simulink model "FTSMC"  (R2022b)
settings: Solver=FixedStepAuto  StartTime=0.0  StopTime=3  FixedStep=1e-5  RelTol=1e-3
libraries: spsSeriesRLCBranchLib x4, spsStairGeneratorLib x3, spsControlledVoltageSourceLib x2, spsCurrentMeasurementLib x2, spsDiodeLib x2, spsIGBTLib x2, spsVariableResistorLib x2, spsVoltageMeasurementLib x2, slpidlib x1, spspowerguiLib x1
settings Model: Creator=10721  LastModifiedBy=10721

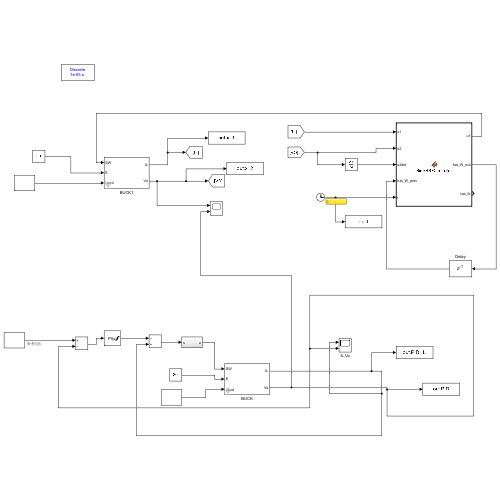
[thumbnail: Simulink's stored preview of the top-level diagram]
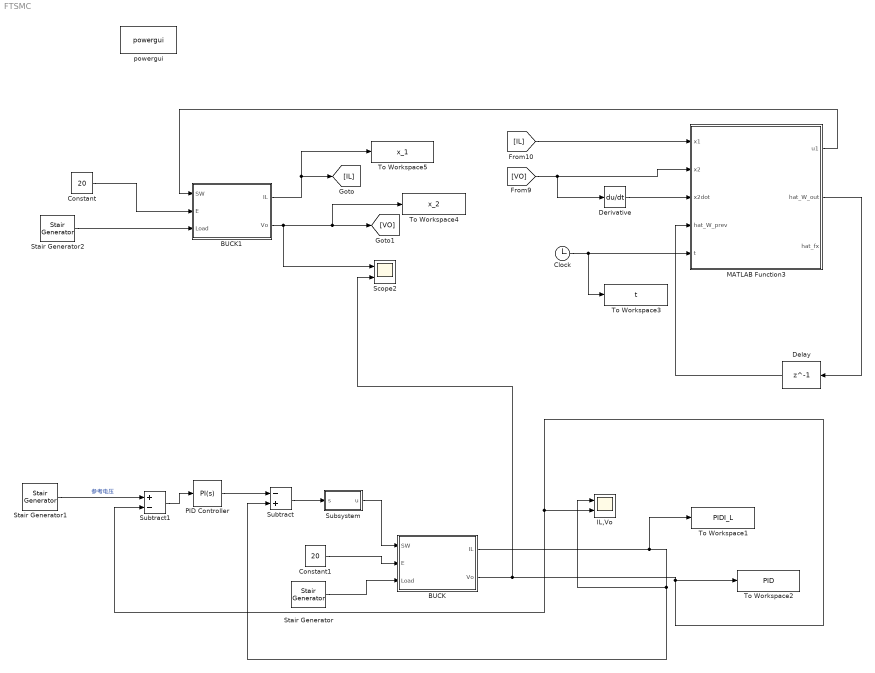
== system FTSMC ==
  BUCK : Subsystem  mask{L=400e-3, C=4e-6}
      mask prompts: L "电感L"; C "电容C"
  BUCK1 : Subsystem  mask{L=100e-3, C=4e-6}
      mask prompts: L "电感L"; C "电容C"
  Clock : Clock
  Constant : Constant  Value=20
  Constant1 : Constant  Value=20
  Delay : Delay  DelayLength=1  InitialCondition=0  UseCircularBuffer=on
  Derivative : Derivative
  IL,Vo : Scope  NumInputPorts=2
  MATLAB Function3 : MATLAB Function  TreatAsAtomicUnit=on
  PID Controller : slpidlib/PID Controller  Controller=PI  Form=Ideal  TimeDomain=Continuous-time  UseExternalTs=off  SampleTime=-1  IntegratorMethod=Forward Euler  FilterMethod=Forward Euler  ControllerParametersSource=internal  P=50  I=10  UseKiTs=off  D=0  N=0  UseFilter=on  TunerSelectOption=Transfer Function Based (PID Tuner App)  InitialConditionSource=internal  InitialConditionForIntegrator=0  InitialConditionForFilter=0  DifferentiatorICPrevScaledInput=0  ExternalReset=none  TrackingMode=off  Kt=1  LimitOutput=on  SatLimitsSource=internal  UpperSaturationLimit=inf  LowerSaturationLimit=-inf  LinearizeAsGain=on  AntiWindupMode=none  Kb=1  LimitIntegrator=off  UpperIntegratorSaturationLimit=inf  LowerIntegratorSaturationLimit=-inf  POutMin=[]  POutMax=[]  IOutMin=[]  IOutMax=[]  DOutMin=[]  DOutMax=[]  NOutMin=[]  NOutMax=[]  SumOutMin=[]  SumOutMax=[]  SaturationOutMin=[]  SaturationOutMax=[]  PParamMin=[]  PParamMax=[]  IParamMin=[]  IParamMax=[]  DParamMin=[]  DParamMax=[]  NParamMin=[]  NParamMax=[]  KbParamMin=[]  KbParamMax=[]  KtParamMin=[]  KtParamMax=[]  KbOutMin=[]  KbOutMax=[]  KtOutMin=[]  KtOutMax=[]  IntegratorOutMin=[]  IntegratorOutMax=[]  FilterOutMin=[]  FilterOutMax=[]  SumI1OutMin=[]  SumI1OutMax=[]  SumI2OutMin=[]  SumI2OutMax=[]  SumI3OutMin=[]  SumI3OutMax=[]  SumI4OutMin=[]  SumI4OutMax=[]  SumDOutMin=[]  SumDOutMax=[]  DifferentiatorOutMin=[]  DifferentiatorOutMax=[]  FilterDiffOutCoefMin=[]  FilterDiffOutCoefMax=[]  ReciprocalOutMin=[]  ReciprocalOutMax=[]  SumDenOutMin=[]  SumDenOutMax=[]  SumNumOutMin=[]  SumNumOutMax=[]  DivideOutMin=[]  DivideOutMax=[]  UdiffTsProdOutMin=[]  UdiffTsProdOutMax=[]  NTsProdOutMin=[]  NTsProdOutMax=[]  UintegralTsProdOutMin=[]  UintegralTsProdOutMax=[]  UngainTsProdOutMin=[]  UngainTsProdOutMax=[]  ClampingZeroOutDataTypeStr=Inherit: Inherit via back propagation  ClampingZeroOutMin=[]  ClampingZeroOutMax=[]  FilterDenConstantOutDataTypeStr=Inherit: Inherit via back propagation  FilterDenConstantOutMin=[]  FilterDenConstantOutMax=[]  PCopyOutDataTypeStr=Inherit: Inherit via back propagation  PCopyOutMin=[]  PCopyOutMax=[]  NCopyOutDataTypeStr=Inherit: Inherit via back propagation  NCopyOutMin=[]  NCopyOutMax=[]  IntegratorContinuousStateAttributes=''  IntegratorStateMustResolveToSignalObject=off  IntegratorRTWStateStorageClass=Auto  FilterContinuousStateAttributes=''  FilterStateMustResolveToSignalObject=off  FilterRTWStateStorageClass=Auto  ParallelPVariant=Passthrough  IdealPVariant=InternalParameters  IVariant=InternalParameters  DVariant=Disabled  IntegratorVariant=Continuous  SatVariant=Enabled  AWVariant=Passthrough  PCopyVariant=Disabled  TRVariant=Disabled  FdbkBlocksVariant=Forward  IdealPFdbkVariant=Disabled  SatFdbkVariant=Disabled  DerivativeFilterVariant=Disabled  NVariant=Disabled  NCopyVariant=Disabled_SignalSpec  FilterICVariant=Disabled  IntegratorICVariant=InternalICs  ExternalResetVariant=Disabled  TRSumVariant=Passthrough  SumFdbkVariant=Disabled  SumVariant=Sum_PI  TsampFilterVariant=InternalTs  TsampNgainVariant=Passthrough  TsampIntegralVariant=Passthrough  ExternalSaturationOutDataTypeStr=Inherit: Same as second input
  Scope2 : Scope  NumInputPorts=2
  Stair Generator : spsStairGeneratorLib/Stair Generator  t="[0  2 ]"  e=[50 55]  Ts=0
  Stair Generator1 : spsStairGeneratorLib/Stair Generator  t=[0 1 ]  e=[10 12 ]  Ts=0
  Stair Generator2 : spsStairGeneratorLib/Stair Generator  t="[0  2 ]"  e=[50 55]  Ts=0
  Subsystem : Subsystem
  Subtract : Sum  Inputs=-+
  Subtract1 : Sum  Inputs=+-
  To Workspace1 : ToWorkspace  VariableName=PIDI_L  SampleTime=-1
  To Workspace2 : ToWorkspace  VariableName=PID  SampleTime=-1
  To Workspace3 : ToWorkspace  VariableName=t  SampleTime=-1
  To Workspace4 : ToWorkspace  VariableName=x_2  SampleTime=-1
  To Workspace5 : ToWorkspace  VariableName=x_1  SampleTime=-1
  powergui : spspowerguiLib/powergui  Priority=1  SimulationMode=Discrete  SampleTime=1e-5  frequency=60  Iterations=50  frequencyindice=0  Pbase=100e6  ErrMax=1e-4  UnitsV=kV  UnitsW=MW  buscounter=0  FunctionMessages=off  echomessages=off  EnableUseOfTLC=off  CurrentSourceSwitches=off  DisableSnubberDevices=off  DisableRonSwitches=off  DisableVfSwitches=off  DisplayEquations=off  AutomaticDiscreteSolvers=off  SolverType=Tustin/Backward Euler (TBE)  Interpol=off  ExternalGateDelay=off  methode=off  Ts=100  x0status=blocks  SPID=on  SwTol=0  HookPort=off  NonlinearTolerance=1e-4  nMaxIteration=100  ContinueOnMaxIteration=off  RestoreLinks=warning  ResistiveCurrentMeasurement=off  Frange=[0:2:500]  Ylog=off  Xlog=on  ShowGrid=off  save=off  variable=ZData  structure=0  ZoomFFT=off  StartTime=0.0  cycles=1  DisplayStyle=1  fundamental=60  FreqAxis=off  MaxFrequency=1000  frequencyindicesteady=1  RmsSteady=1  display=off
  wires:
  Constant/1 -> BUCK1/2(E)
  BUCK1/1(IL) -> To Workspace5/1, [IL]
  Stair Generator2/1 -> BUCK1/3(Load)
  BUCK1/2(Vo) -> Scope2/1, To Workspace4/1, [VO]
  [IL] -> MATLAB Function3/1(x1)
  Clock/1 -> MATLAB Function3/5(t), To Workspace3/1
  [VO] -> Derivative/1, MATLAB Function3/2(x2)
  MATLAB Function3/2(hat_W_out) -> Delay/1
  MATLAB Function3/1(u1) -> BUCK1/1(SW)
  Delay/1 -> MATLAB Function3/4(hat_W_prev)
  Stair Generator1/1 -> Subtract1/1  "参考电压"
  Subsystem/1(u) -> BUCK/1(SW)
  Stair Generator/1 -> BUCK/3(Load)
  BUCK/2(Vo) -> Scope2/2, IL,Vo/2, Subtract1/2, To Workspace2/1
  Constant1/1 -> BUCK/2(E)
  BUCK/1(IL) -> To Workspace1/1, IL,Vo/1, Subtract/2
  PID Controller/1 -> Subtract/1
  Subtract/1 -> Subsystem/1(s)
  Subtract1/1 -> PID Controller/1
  Derivative/1 -> MATLAB Function3/3(x2dot)

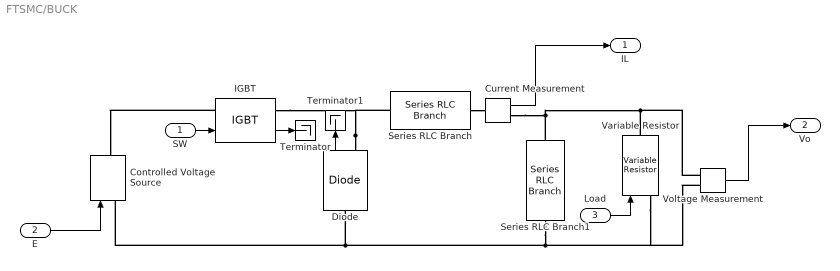
== system FTSMC/BUCK ==
  SW : Inport
  E : Inport  Port=2
  Load : Inport  Port=3
  Controlled Voltage Source : spsControlledVoltageSourceLib/Controlled Voltage Source  Initialize=on  Source_Type=AC  Amplitude=0  Phase=0  Frequency=0  Measurements=None
  Current Measurement : spsCurrentMeasurementLib/Current Measurement  PhasorSimulation=off  OutputType=Complex  PSBequivalent=0
  Diode : spsDiodeLib/Diode  Ron=0.001  Lon=0  Vf=0.8  IC=0  UseSnubber=0  Rs=500  Cs=250e-9  Measurements=on
  IGBT : spsIGBTLib/IGBT  Ron=0.001  Lon=0  Vf=1  Tf=1e-6  Tt=2e-6  IC=0  Rs=1e5  Cs=inf  Measurements=on
  Series RLC Branch : spsSeriesRLCBranchLib/Series RLC Branch  LConnTagsString=__new0  RConnTagsString=__new0  BranchType=L  Resistance=1  Inductance=L  SetiL0=off  InitialCurrent=0  Capacitance=1e-6  Setx0=off  InitialVoltage=0  Measurements=None
  Series RLC Branch1 : spsSeriesRLCBranchLib/Series RLC Branch  LConnTagsString=__new0  RConnTagsString=__new0  BranchType=C  Resistance=1  Inductance=1e-3  SetiL0=off  InitialCurrent=0  Capacitance=C  Setx0=off  InitialVoltage=0  Measurements=None
  Terminator : Terminator
  Terminator1 : Terminator
  Variable Resistor : spsVariableResistorLib/Variable Resistor  Rabsmin=1e-3
  Voltage Measurement : spsVoltageMeasurementLib/Voltage Measurement  PhasorSimulation=off  OutputType=Complex  PSBequivalent=0
  IL : Outport
  Vo : Outport  Port=2
  wires:
  Load/1 -> Variable Resistor/1
  E/1 -> Controlled Voltage Source/1
  Voltage Measurement/1 -> Vo/1
  SW/1 -> IGBT/1
  Diode/1 -> Terminator1/1
  IGBT/1 -> Terminator/1
  Current Measurement/1 -> IL/1
  connections:
  Current Measurement/RConn1 -- Variable Resistor/RConn1 -- Voltage Measurement/LConn1 -- Series RLC Branch1/LConn1
  IGBT/LConn1 -- Controlled Voltage Source/RConn1
  Series RLC Branch1/RConn1 -- Variable Resistor/LConn1 -- Voltage Measurement/LConn2 -- Controlled Voltage Source/LConn1 -- Diode/LConn1
  Series RLC Branch/RConn1 -- Current Measurement/LConn1
  Diode/RConn1 -- Series RLC Branch/LConn1 -- IGBT/RConn1

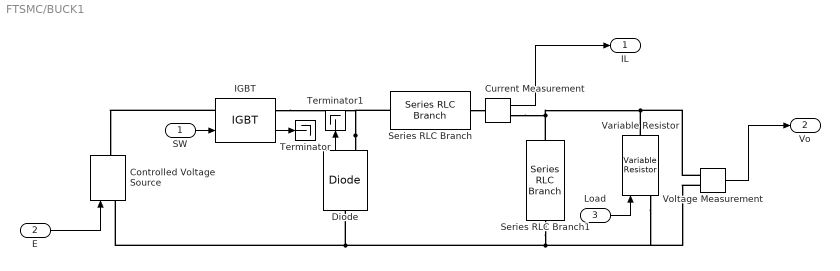
== system FTSMC/BUCK1 ==
  SW : Inport
  E : Inport  Port=2
  Load : Inport  Port=3
  Controlled Voltage Source : spsControlledVoltageSourceLib/Controlled Voltage Source  Initialize=on  Source_Type=AC  Amplitude=0  Phase=0  Frequency=0  Measurements=None
  Current Measurement : spsCurrentMeasurementLib/Current Measurement  PhasorSimulation=off  OutputType=Complex  PSBequivalent=0
  Diode : spsDiodeLib/Diode  Ron=0.001  Lon=0  Vf=0.8  IC=0  UseSnubber=0  Rs=500  Cs=250e-9  Measurements=on
  IGBT : spsIGBTLib/IGBT  Ron=0.001  Lon=0  Vf=1  Tf=1e-6  Tt=2e-6  IC=0  Rs=1e5  Cs=inf  Measurements=on
  Series RLC Branch : spsSeriesRLCBranchLib/Series RLC Branch  LConnTagsString=__new0  RConnTagsString=__new0  BranchType=L  Resistance=1  Inductance=L  SetiL0=off  InitialCurrent=0  Capacitance=1e-6  Setx0=off  InitialVoltage=0  Measurements=None
  Series RLC Branch1 : spsSeriesRLCBranchLib/Series RLC Branch  LConnTagsString=__new0  RConnTagsString=__new0  BranchType=C  Resistance=1  Inductance=1e-3  SetiL0=off  InitialCurrent=0  Capacitance=C  Setx0=off  InitialVoltage=0  Measurements=None
  Terminator : Terminator
  Terminator1 : Terminator
  Variable Resistor : spsVariableResistorLib/Variable Resistor  Rabsmin=1e-3
  Voltage Measurement : spsVoltageMeasurementLib/Voltage Measurement  PhasorSimulation=off  OutputType=Complex  PSBequivalent=0
  IL : Outport
  Vo : Outport  Port=2
  wires:
  Load/1 -> Variable Resistor/1
  E/1 -> Controlled Voltage Source/1
  Voltage Measurement/1 -> Vo/1
  SW/1 -> IGBT/1
  Diode/1 -> Terminator1/1
  IGBT/1 -> Terminator/1
  Current Measurement/1 -> IL/1
  connections:
  Current Measurement/RConn1 -- Variable Resistor/RConn1 -- Voltage Measurement/LConn1 -- Series RLC Branch1/LConn1
  IGBT/LConn1 -- Controlled Voltage Source/RConn1
  Series RLC Branch1/RConn1 -- Variable Resistor/LConn1 -- Voltage Measurement/LConn2 -- Controlled Voltage Source/LConn1 -- Diode/LConn1
  Series RLC Branch/RConn1 -- Current Measurement/LConn1
  Diode/RConn1 -- Series RLC Branch/LConn1 -- IGBT/RConn1

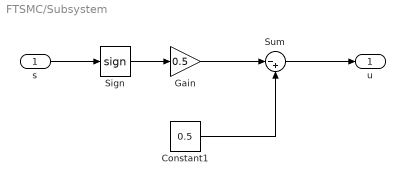
== system FTSMC/Subsystem ==
  s : Inport
  Constant1 : Constant  Value=0.5
  Gain : Gain  Gain=0.5
  Sign : Signum
  Sum : Sum  Inputs=|-+
  u : Outport
  wires:
  Gain/1 -> Sum/1
  s/1 -> Sign/1
  Sum/1 -> u/1
  Sign/1 -> Gain/1
  Constant1/1 -> Sum/2

== matlab function FTSMC/MATLAB Function3 ==
  settings: updateMethod=DISCRETE
  data: u1 output; hat_W_out output; x1 input; hat_fx output; x2 input; x2dot input; hat_W_prev input; t input
function [u1, hat_W_out, hat_fx] = BuckRBFController(x1, x2,x2dot, hat_W_prev, t)



coder.varsize('u1', [1, 1], [0, 0]);
coder.varsize('hat_W_out', [5, 1], [0, 0]);
coder.varsize('hat_fx', [1, 1], [0, 0]);
coder.varsize('e_out', [1, 1], [0, 0]);
coder.varsize('s_out', [1, 1], [0, 0]);


u1 = 0;
hat_W_out = zeros(5, 1);
hat_fx = 0;
e_out = 0;
s_out = 0;


L = 100e-3;    
C = 4e-6;    
E = 20;       


b = 20;
c = 15000;
c1 = 10000;
b1 = 10000;


gamma = 500;
dT = 0.00001;


c_i = [-2 -1  0  1  1; 
       -2 -1  0  1  1];
b_i = 0.9;


if t <= 1
    x2d = 10;  
else
    x2d = 12;  
end
dot_x2d = 0;
e = x2 - x2d;
dot_e = x2dot;  

if e >= 0
    s = b * e + dot_e + c * (abs(e)^0.25);
else
    s = b * e + dot_e - c * (abs(e)^0.25);
end

h = zeros(5, 1);
input = [x1; x2];

for i = 1:5
    diff = input - c_i(:, i);
    distance_sq = diff(1)^2 + diff(2)^2;
    h(i) = exp(-distance_sq / (2 * b_i^2));
end


hat_fx = hat_W_prev' * h;


hat_W_out = hat_W_prev + dT * gamma * s * h;


u1 = (C * L / E) * ((1/(C*L)))*x2+hat_fx-b*dot_e-(c/4)*(abs(e))^(-0.75)*dot_e-c1*sign(s)-b1*s;              


if u1 > 1
    u1 = 1;
elseif u1 < 0
    u1 = 0;
end


end
